simulink model "L400_plant"  (R2022b)
settings: Solver=VariableStepAuto  StartTime=0.0  StopTime=10.0  RelTol=1e-3
InitFcn:
  | L400_init
values from neighbouring files (symbols this model uses):
  db = read_aerody_base('L400气动力数据库.V1.20241219.txt')    [plot_aerody_base.m]
undefined symbols (not defined in the file or in its folder): Earth, Im0, Jm, Kd, Ke, Lm, Rm, WGS84
libraries: aerolibasang x2, aerolib6dof2 x1, matrix_library x1
settings Model: Creator=CETCA  LastModifiedBy=CETCA

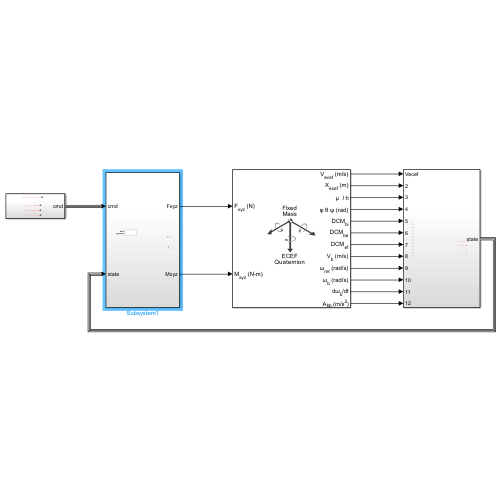
[thumbnail: Simulink's stored preview of the top-level diagram]
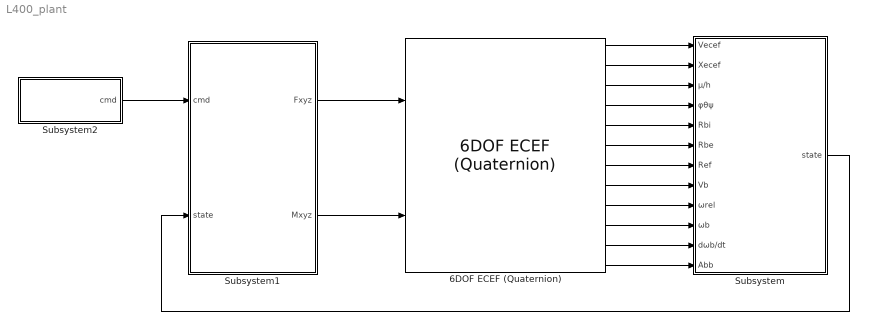
== system L400_plant ==
  6DOF ECEF (Quaternion) : aerolib6dof2/6DOF ECEF (Quaternion)  units=Metric (MKS)  mtype=Fixed  xg_0=[0 0 0]  Vm_0=[0 0 0]  eul_0=[0 0 0]  pm_0=[0 0 0]  mass_0=1.0  mass_e=0.5  mass_f=2.0  inertia=eye(3)  inertia_e=eye(3)  inertia_f=2*eye(3)  vre_flag=on  abi_flag=off  ptype=Earth (WGS84)  R=6378137  F=1/298.257223563  w_E=7292115e-11  angle_in=Internal  LG0=0  quat_statename=''  pm_statename=''  Vm_statename=''  posECEF_statename=''  posECI_statename=''  LG_statename=''  mass_statename=''
  Subsystem : Subsystem
  Subsystem1 : Subsystem
  Subsystem2 : Subsystem
  wires:
  Subsystem/1(state) -> Subsystem1/2(state)
  Subsystem1/1(Fxyz) -> 6DOF ECEF (Quaternion)/1
  Subsystem1/2(Mxyz) -> 6DOF ECEF (Quaternion)/2
  Subsystem2/1(cmd) -> Subsystem1/1(cmd)
  6DOF ECEF (Quaternion)/1 -> Subsystem/1(Vecef)
  6DOF ECEF (Quaternion)/2 -> Subsystem/2(Xecef)
  6DOF ECEF (Quaternion)/3 -> Subsystem/3(μ/h)
  6DOF ECEF (Quaternion)/4 -> Subsystem/4(φθψ)
  6DOF ECEF (Quaternion)/5 -> Subsystem/5(Rbi)
  6DOF ECEF (Quaternion)/6 -> Subsystem/6(Rbe)
  6DOF ECEF (Quaternion)/7 -> Subsystem/7(Ref)
  6DOF ECEF (Quaternion)/8 -> Subsystem/8(Vb)
  6DOF ECEF (Quaternion)/9 -> Subsystem/9(ωrel)
  6DOF ECEF (Quaternion)/10 -> Subsystem/10(ωb)
  6DOF ECEF (Quaternion)/11 -> Subsystem/11(dωb/dt)
  6DOF ECEF (Quaternion)/12 -> Subsystem/12(Abb)

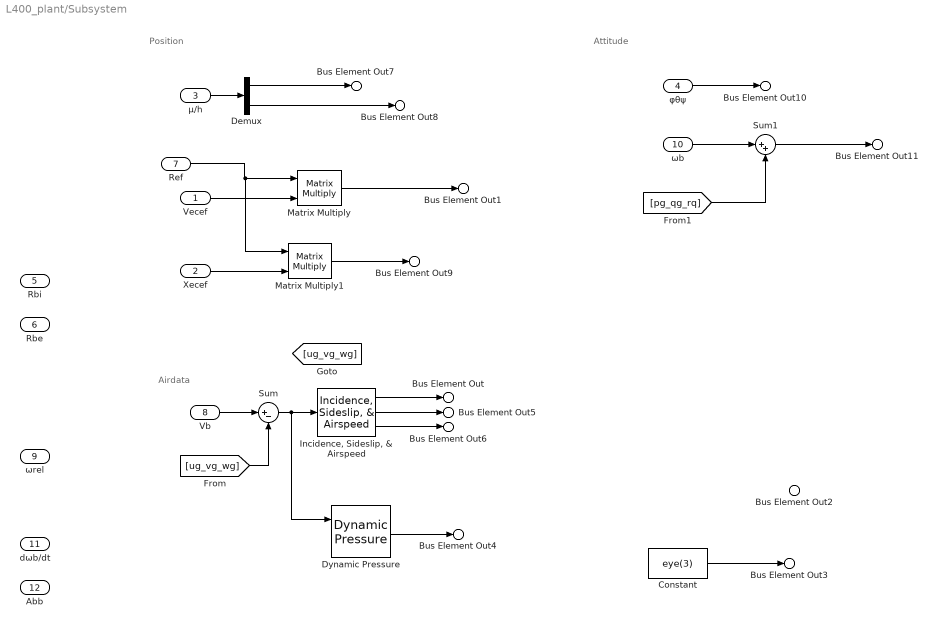
== system L400_plant/Subsystem ==
  note: Attitude
  note: Airdata
  note: Position
  Vecef : Inport
  Xecef : Inport  Port=2
  μ/h : Inport  Port=3
  φθψ : Inport  Port=4
  Rbi : Inport  Port=5
  Rbe : Inport  Port=6
  Ref : Inport  Port=7
  Vb : Inport  Port=8
  ωrel : Inport  Port=9
  ωb : Inport  Port=10
  dωb/dt : Inport  Port=11
  Abb : Inport  Port=12
  Constant : Constant  Value=eye(3)
  Demux : Demux  Outputs=[2 1]
  Dynamic Pressure : aerolibasang/Dynamic Pressure
  "Incidence, Sideslip, & Airspeed" : aerolibasang/Incidence, Sideslip, & Airspeed
  Matrix Multiply : Product  Multiplication=Matrix(*)
  Matrix Multiply1 : Product  Multiplication=Matrix(*)
  Sum : Sum  Inputs=|+-
  Sum1 : Sum  Inputs=|++
  Bus Element Out : Outport  PortName=state  Element=alpha
  Bus Element Out1 : Outport  PortName=state  Element=vn_ve_vd
  Bus Element Out2 : Outport  PortName=state  Element=height
  Bus Element Out3 : Outport  PortName=state  Element=Rbw
  Bus Element Out4 : Outport  PortName=state  Element=qbar
  Bus Element Out5 : Outport  PortName=state  Element=beta
  Bus Element Out6 : Outport  PortName=state  Element=airspeed
  Bus Element Out7 : Outport  PortName=state  Element=lat_lon
  Bus Element Out8 : Outport  PortName=state  Element=alt
  Bus Element Out9 : Outport  PortName=state  Element=pn_pe_pd
  Bus Element Out10 : Outport  PortName=state  Element=phi_theta_psi
  Bus Element Out11 : Outport  PortName=state  Element=p_q_r
  wires:
  Matrix Multiply/1 -> Bus Element Out1/1
  "Incidence, Sideslip, & Airspeed"/1 -> Bus Element Out/1
  Constant/1 -> Bus Element Out3/1
  Vecef/1 -> Matrix Multiply/2
  Ref/1 -> Matrix Multiply1/1, Matrix Multiply/1
  Vb/1 -> Sum/1
  Sum/1 -> Dynamic Pressure/1, "Incidence, Sideslip, & Airspeed"/1
  "Incidence, Sideslip, & Airspeed"/2 -> Bus Element Out5/1
  "Incidence, Sideslip, & Airspeed"/3 -> Bus Element Out6/1
  [ug_vg_wg] -> Sum/2
  Dynamic Pressure/1 -> Bus Element Out4/1
  μ/h/1 -> Demux/1
  Demux/1 -> Bus Element Out7/1
  Demux/2 -> Bus Element Out8/1
  Xecef/1 -> Matrix Multiply1/2
  Matrix Multiply1/1 -> Bus Element Out9/1
  φθψ/1 -> Bus Element Out10/1
  ωb/1 -> Sum1/1
  Sum1/1 -> Bus Element Out11/1
  [pg_qg_rq] -> Sum1/2

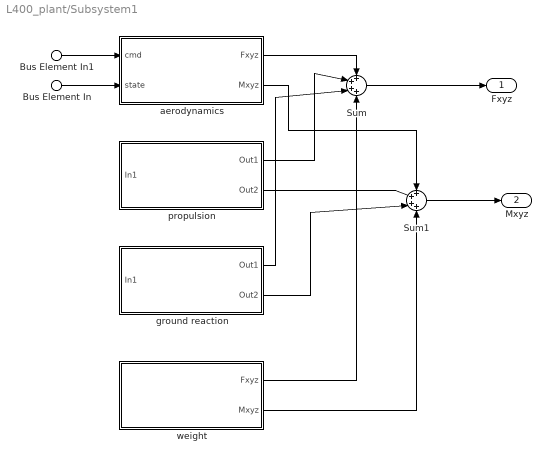
== system L400_plant/Subsystem1 ==
  Bus Element In1 : Inport  PortName=cmd
  Bus Element In : Inport  Port=2  PortName=state
  Sum : Sum  Inputs=4
  Sum1 : Sum  Inputs=4
  aerodynamics : Subsystem
  ground reaction : Subsystem
  propulsion : Subsystem
  weight : Subsystem
  Fxyz : Outport
  Mxyz : Outport  Port=2
  wires:
  Bus Element In/1 -> aerodynamics/2(state)
  Bus Element In1/1 -> aerodynamics/1(cmd)
  propulsion/2(Out2) -> Sum1/2
  aerodynamics/1(Fxyz) -> Sum/1
  propulsion/1(Out1) -> Sum/2
  aerodynamics/2(Mxyz) -> Sum1/1
  Sum1/1 -> Mxyz/1
  Sum/1 -> Fxyz/1
  ground reaction/1(Out1) -> Sum/3
  ground reaction/2(Out2) -> Sum1/3
  weight/1(Fxyz) -> Sum/4
  weight/2(Mxyz) -> Sum1/4

== system L400_plant/Subsystem2 ==
  Bus Element Out : Outport  PortName=cmd  Element=df
  Bus Element Out1 : Outport  PortName=cmd  Element=da
  Bus Element Out2 : Outport  PortName=cmd  Element=dr
  Bus Element Out3 : Outport  PortName=cmd  Element=de
  wires:
  ? -> Bus Element Out/1
  ? -> Bus Element Out1/1
  ? -> Bus Element Out3/1
  ? -> Bus Element Out2/1

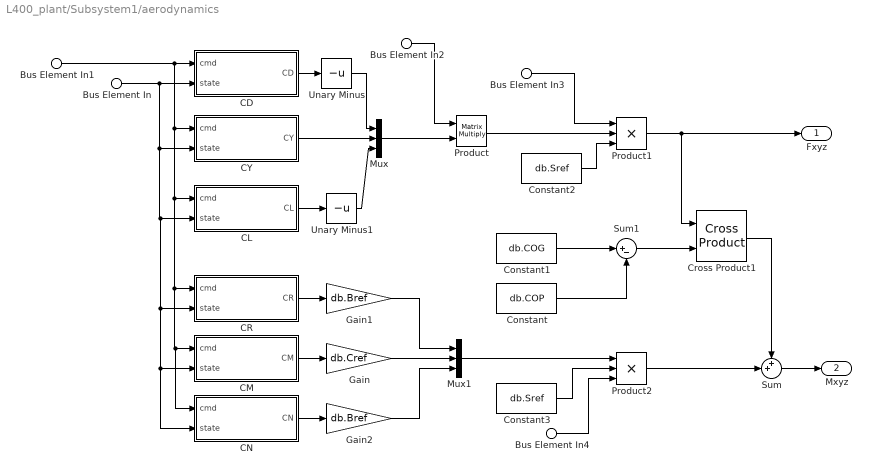
== system L400_plant/Subsystem1/aerodynamics ==
  Bus Element In1 : Inport  PortName=cmd
  Bus Element In : Inport  Port=2  PortName=state
  Bus Element In2 : Inport  Port=2  PortName=state  Element=Rbw
  Bus Element In3 : Inport  Port=2  PortName=state  Element=qbar
  Bus Element In4 : Inport  Port=2  PortName=state  Element=qbar
  CD : Subsystem
  CL : Subsystem
  CM : Subsystem
  CN : Subsystem
  CR : Subsystem
  CY : Subsystem
  Constant : Constant  Value=db.COP
  Constant1 : Constant  Value=db.COG
  Constant2 : Constant  Value=db.Sref
  Constant3 : Constant  Value=db.Sref
  Cross Product1 : matrix_library/Cross Product
  Gain : Gain  Gain=db.Cref
  Gain1 : Gain  Gain=db.Bref
  Gain2 : Gain  Gain=db.Bref
  Mux : Mux  Inputs=3
  Mux1 : Mux  Inputs=3
  Product : Product  Multiplication=Matrix(*)
  Product1 : Product  Inputs=3
  Product2 : Product  Inputs=3
  Sum : Sum  Inputs=++|
  Sum1 : Sum  Inputs=|+-
  Unary Minus : UnaryMinus
  Unary Minus1 : UnaryMinus
  Fxyz : Outport
  Mxyz : Outport  Port=2
  wires:
  Bus Element In1/1 -> CN/1(cmd), CM/1(cmd), CR/1(cmd), CL/1(cmd), CY/1(cmd), CD/1(cmd)
  Bus Element In/1 -> CN/2(state), CM/2(state), CR/2(state), CL/2(state), CY/2(state), CD/2(state)
  Mux/1 -> Product/2
  CD/1(CD) -> Unary Minus/1
  CY/1(CY) -> Mux/2
  CL/1(CL) -> Unary Minus1/1
  Unary Minus/1 -> Mux/1
  Unary Minus1/1 -> Mux/3
  Product/1 -> Product1/2
  Bus Element In2/1 -> Product/1
  CM/1(CM) -> Gain/1
  CR/1(CR) -> Gain1/1
  CN/1(CN) -> Gain2/1
  Mux1/1 -> Product2/1
  Sum/1 -> Mxyz/1
  Cross Product1/1 -> Sum/1
  Constant1/1 -> Sum1/1
  Constant/1 -> Sum1/2
  Product1/1 -> Cross Product1/1, Fxyz/1
  Bus Element In3/1 -> Product1/1
  Constant2/1 -> Product1/3
  Product2/1 -> Sum/2
  Bus Element In4/1 -> Product2/3
  Constant3/1 -> Product2/2
  Gain/1 -> Mux1/2
  Gain1/1 -> Mux1/1
  Gain2/1 -> Mux1/3
  Sum1/1 -> Cross Product1/2

== system L400_plant/Subsystem1/ground reaction ==
  In1 : Inport
  Out1 : Outport
  Out2 : Outport  Port=2

== system L400_plant/Subsystem1/propulsion ==
  In1 : Inport
  Subsystem : Subsystem
  Out1 : Outport
  Out2 : Outport  Port=2

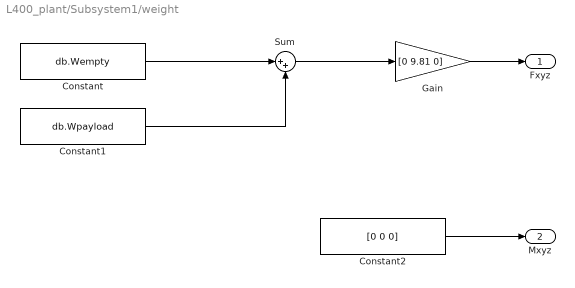
== system L400_plant/Subsystem1/weight ==
  Constant : Constant  Value=db.Wempty
  Constant1 : Constant  Value=db.Wpayload
  Constant2 : Constant  Value=[0 0 0]
  Gain : Gain  Gain=[0 9.81 0]
  Sum : Sum  Inputs=|++
  Fxyz : Outport
  Mxyz : Outport  Port=2
  wires:
  Constant/1 -> Sum/1
  Constant1/1 -> Sum/2
  Sum/1 -> Gain/1
  Gain/1 -> Fxyz/1
  Constant2/1 -> Mxyz/1

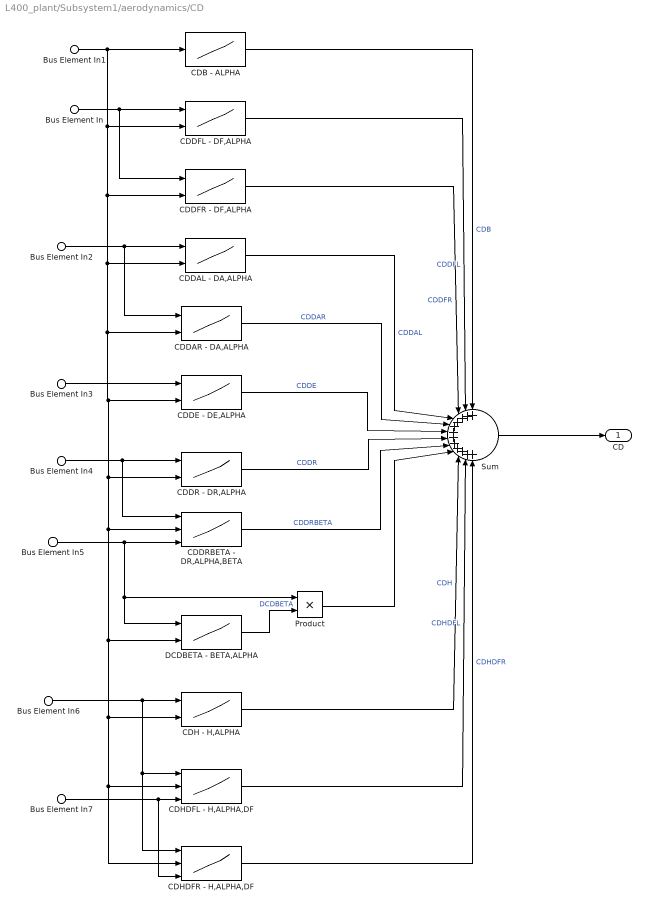
== system L400_plant/Subsystem1/aerodynamics/CD ==
  Bus Element In : Inport  PortName=cmd  Element=df
  Bus Element In7 : Inport  PortName=cmd  Element=df
  Bus Element In2 : Inport  PortName=cmd  Element=da
  Bus Element In3 : Inport  PortName=cmd  Element=de
  Bus Element In4 : Inport  PortName=cmd  Element=dr
  Bus Element In1 : Inport  Port=2  PortName=state  Element=alpha
  Bus Element In5 : Inport  Port=2  PortName=state  Element=vn_ve_vd
  Bus Element In6 : Inport  Port=2  PortName=state  Element=height
  CDB - ALPHA : Lookup_n-D  NumberOfTableDimensions=1  BreakpointsForDimension1=db.VALPHA  Table=db.CDB  InternalRulePriority=Speed  RndMeth=Simplest
  CDDAL - DA,ALPHA : Lookup_n-D  BreakpointsForDimension1=db.VDA  BreakpointsForDimension2=db.VALPHA  Table=db.CDDAL  InternalRulePriority=Speed  RndMeth=Simplest
      settings: InputPortMap=u0,u1
  CDDAR - DA,ALPHA : Lookup_n-D  BreakpointsForDimension1=db.VDA  BreakpointsForDimension2=db.VALPHA  Table=db.CDDAR  InternalRulePriority=Speed  RndMeth=Simplest
      settings: InputPortMap=u0,u1
  CDDE - DE,ALPHA : Lookup_n-D  BreakpointsForDimension1=db.VDE  BreakpointsForDimension2=db.VALPHA  Table=db.CDDE  InternalRulePriority=Speed  RndMeth=Simplest
      settings: InputPortMap=u0,u1
  CDDFL - DF,ALPHA : Lookup_n-D  BreakpointsForDimension1=db.VDF  BreakpointsForDimension2=db.VALPHA  Table=db.CDDFL  InternalRulePriority=Speed  RndMeth=Simplest
      settings: InputPortMap=u0,u1
  CDDFR - DF,ALPHA : Lookup_n-D  BreakpointsForDimension1=db.VDF  BreakpointsForDimension2=db.VALPHA  Table=db.CDDFR  InternalRulePriority=Speed  RndMeth=Simplest
      settings: InputPortMap=u0,u1
  CDDR - DR,ALPHA : Lookup_n-D  BreakpointsForDimension1=db.VDR  BreakpointsForDimension2=db.VALPHA  Table=db.CDDR  InternalRulePriority=Speed  RndMeth=Simplest
      settings: InputPortMap=u0,u1
  CDDRBETA - DR,ALPHA,BETA : Lookup_n-D  NumberOfTableDimensions=3  BreakpointsForDimension1=db.VDR  BreakpointsForDimension2=db.VALPHA  BreakpointsForDimension3=db.VBETA  Table=db.CDDRBETA  InternalRulePriority=Speed  RndMeth=Simplest
      settings: InputPortMap=u0,u1,u2
  CDH - H,ALPHA : Lookup_n-D  BreakpointsForDimension1=db.VH  BreakpointsForDimension2=db.VALPHA  Table=db.CDH  InternalRulePriority=Speed  RndMeth=Simplest
      settings: InputPortMap=u0,u1
  CDHDFL - H,ALPHA,DF : Lookup_n-D  NumberOfTableDimensions=3  BreakpointsForDimension1=db.VH  BreakpointsForDimension2=db.VALPHA  BreakpointsForDimension3=db.VDF  Table=db.CDHDFL  InternalRulePriority=Speed  RndMeth=Simplest
      settings: InputPortMap=u0,u1,u2
  CDHDFR - H,ALPHA,DF : Lookup_n-D  NumberOfTableDimensions=3  BreakpointsForDimension1=db.VH  BreakpointsForDimension2=db.VALPHA  BreakpointsForDimension3=db.VDF  Table=db.CDHDFR  InternalRulePriority=Speed  RndMeth=Simplest
      settings: InputPortMap=u0,u1,u2
  DCDBETA - BETA,ALPHA : Lookup_n-D  BreakpointsForDimension1=db.VBETA  BreakpointsForDimension2=db.VALPHA  Table=db.DCDBETA  InternalRulePriority=Speed  RndMeth=Simplest
      settings: InputPortMap=u0,u1
  Product : Product
  Sum : Sum  Inputs=12
  CD : Outport
  wires:
  CDB - ALPHA/1 -> Sum/1  "CDB"
  Bus Element In1/1 -> CDDAR - DA,ALPHA/2, CDDR - DR,ALPHA/2, CDDRBETA - DR,ALPHA,BETA/2, DCDBETA - BETA,ALPHA/2, CDHDFL - H,ALPHA,DF/2, CDHDFR - H,ALPHA,DF/2, CDH - H,ALPHA/2, CDDE - DE,ALPHA/2, CDDAL - DA,ALPHA/2, CDDFR - DF,ALPHA/2, CDDFL - DF,ALPHA/2, CDB - ALPHA/1
  CDDFL - DF,ALPHA/1 -> Sum/2  "CDDFL"
  Bus Element In/1 -> CDDFR - DF,ALPHA/1, CDDFL - DF,ALPHA/1
  CDDFR - DF,ALPHA/1 -> Sum/3  "CDDFR"
  CDDAL - DA,ALPHA/1 -> Sum/4  "CDDAL"
  Bus Element In2/1 -> CDDAR - DA,ALPHA/1, CDDAL - DA,ALPHA/1
  CDDAR - DA,ALPHA/1 -> Sum/5  "CDDAR"
  CDDE - DE,ALPHA/1 -> Sum/6  "CDDE"
  Bus Element In3/1 -> CDDE - DE,ALPHA/1
  CDDR - DR,ALPHA/1 -> Sum/7  "CDDR"
  Bus Element In4/1 -> CDDRBETA - DR,ALPHA,BETA/1, CDDR - DR,ALPHA/1
  CDDRBETA - DR,ALPHA,BETA/1 -> Sum/8  "CDDRBETA"
  Bus Element In5/1 -> Product/1, DCDBETA - BETA,ALPHA/1, CDDRBETA - DR,ALPHA,BETA/3
  DCDBETA - BETA,ALPHA/1 -> Product/2  "DCDBETA"
  Product/1 -> Sum/9
  CDH - H,ALPHA/1 -> Sum/10  "CDH"
  Bus Element In6/1 -> CDHDFR - H,ALPHA,DF/1, CDHDFL - H,ALPHA,DF/1, CDH - H,ALPHA/1
  CDHDFL - H,ALPHA,DF/1 -> Sum/11  "CDHDFL"
  Bus Element In7/1 -> CDHDFR - H,ALPHA,DF/3, CDHDFL - H,ALPHA,DF/3
  CDHDFR - H,ALPHA,DF/1 -> Sum/12  "CDHDFR"
  Sum/1 -> CD/1

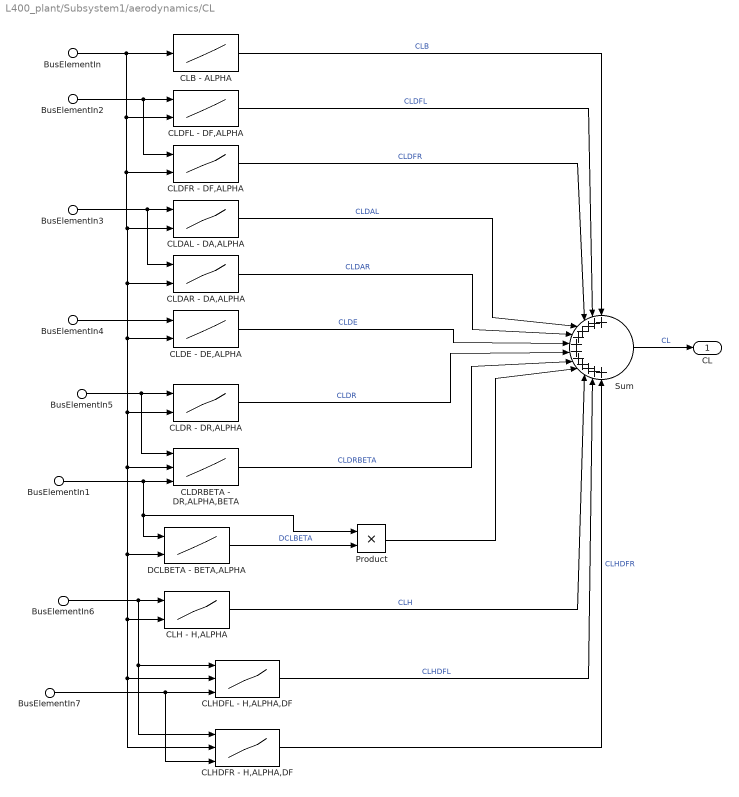
== system L400_plant/Subsystem1/aerodynamics/CL ==
  BusElementIn2 : Inport  PortName=cmd  Element=df
  BusElementIn7 : Inport  PortName=cmd  Element=df
  BusElementIn3 : Inport  PortName=cmd  Element=da
  BusElementIn4 : Inport  PortName=cmd  Element=de
  BusElementIn5 : Inport  PortName=cmd  Element=dr
  BusElementIn : Inport  Port=2  PortName=state  Element=alpha
  BusElementIn1 : Inport  Port=2  PortName=state  Element=vn_ve_vd
  BusElementIn6 : Inport  Port=2  PortName=state  Element=height
  CLB - ALPHA : Lookup_n-D  NumberOfTableDimensions=1  BreakpointsForDimension1=db.VALPHA  Table=db.CLB  InternalRulePriority=Speed  RndMeth=Simplest
  CLDAL - DA,ALPHA : Lookup_n-D  BreakpointsForDimension1=db.VDA  BreakpointsForDimension2=db.VALPHA  Table=db.CLDAL  InternalRulePriority=Speed  RndMeth=Simplest
      settings: InputPortMap=u0,u1
  CLDAR - DA,ALPHA : Lookup_n-D  BreakpointsForDimension1=db.VDA  BreakpointsForDimension2=db.VALPHA  Table=db.CLDAR  InternalRulePriority=Speed  RndMeth=Simplest
      settings: InputPortMap=u0,u1
  CLDE - DE,ALPHA : Lookup_n-D  BreakpointsForDimension1=db.VDE  BreakpointsForDimension2=db.VALPHA  Table=db.CLDE  InternalRulePriority=Speed  RndMeth=Simplest
      settings: InputPortMap=u0,u1
  CLDFL - DF,ALPHA : Lookup_n-D  BreakpointsForDimension1=db.VDF  BreakpointsForDimension2=db.VALPHA  Table=db.CLDFL  InternalRulePriority=Speed  RndMeth=Simplest
      settings: InputPortMap=u0,u1
  CLDFR - DF,ALPHA : Lookup_n-D  BreakpointsForDimension1=db.VDF  BreakpointsForDimension2=db.VALPHA  Table=db.CLDFR  InternalRulePriority=Speed  RndMeth=Simplest
      settings: InputPortMap=u0,u1
  CLDR - DR,ALPHA : Lookup_n-D  BreakpointsForDimension1=db.VDR  BreakpointsForDimension2=db.VALPHA  Table=db.CLDR  InternalRulePriority=Speed  RndMeth=Simplest
      settings: InputPortMap=u0,u1
  CLDRBETA - DR,ALPHA,BETA : Lookup_n-D  NumberOfTableDimensions=3  BreakpointsForDimension1=db.VDR  BreakpointsForDimension2=db.VALPHA  BreakpointsForDimension3=db.VBETA  Table=db.CLDRBETA  InternalRulePriority=Speed  RndMeth=Simplest
      settings: InputPortMap=u0,u1,u2
  CLH - H,ALPHA : Lookup_n-D  BreakpointsForDimension1=db.VH  BreakpointsForDimension2=db.VALPHA  BreakpointsForDimension3=db.VBETA  Table=db.CLH  InternalRulePriority=Speed  RndMeth=Simplest
      settings: InputPortMap=u0,u1
  CLHDFL - H,ALPHA,DF : Lookup_n-D  NumberOfTableDimensions=3  BreakpointsForDimension1=db.VH  BreakpointsForDimension2=db.VALPHA  BreakpointsForDimension3=db.VDF  Table=db.CLHDFL  InternalRulePriority=Speed  RndMeth=Simplest
      settings: InputPortMap=u0,u1,u2
  CLHDFR - H,ALPHA,DF : Lookup_n-D  NumberOfTableDimensions=3  BreakpointsForDimension1=db.VH  BreakpointsForDimension2=db.VALPHA  BreakpointsForDimension3=db.VDF  Table=db.CLHDFL  InternalRulePriority=Speed  RndMeth=Simplest
      settings: InputPortMap=u0,u1,u2
  DCLBETA - BETA,ALPHA : Lookup_n-D  BreakpointsForDimension1=db.VBETA  BreakpointsForDimension2=db.VALPHA  BreakpointsForDimension3=db.VBETA  Table=db.DCLBETA  InternalRulePriority=Speed  RndMeth=Simplest
      settings: InputPortMap=u0,u1
  Product : Product
  Sum : Sum  Inputs=12
  CL : Outport
  wires:
  BusElementIn/1 -> DCLBETA - BETA,ALPHA/2, CLHDFR - H,ALPHA,DF/2, CLHDFL - H,ALPHA,DF/2, CLH - H,ALPHA/2, CLDRBETA - DR,ALPHA,BETA/2, CLDR - DR,ALPHA/2, CLDE - DE,ALPHA/2, CLDAR - DA,ALPHA/2, CLDAL - DA,ALPHA/2, CLDFR - DF,ALPHA/2, CLDFL - DF,ALPHA/2, CLB - ALPHA/1
  CLB - ALPHA/1 -> Sum/1  "CLB"
  BusElementIn2/1 -> CLDFR - DF,ALPHA/1, CLDFL - DF,ALPHA/1
  CLDFL - DF,ALPHA/1 -> Sum/2  "CLDFL"
  CLDFR - DF,ALPHA/1 -> Sum/3  "CLDFR"
  CLDAL - DA,ALPHA/1 -> Sum/4  "CLDAL"
  BusElementIn3/1 -> CLDAR - DA,ALPHA/1, CLDAL - DA,ALPHA/1
  CLDAR - DA,ALPHA/1 -> Sum/5  "CLDAR"
  BusElementIn4/1 -> CLDE - DE,ALPHA/1
  CLDE - DE,ALPHA/1 -> Sum/6  "CLDE"
  CLDR - DR,ALPHA/1 -> Sum/7  "CLDR"
  BusElementIn5/1 -> CLDRBETA - DR,ALPHA,BETA/1, CLDR - DR,ALPHA/1
  Sum/1 -> CL/1  "CL"
  CLDRBETA - DR,ALPHA,BETA/1 -> Sum/8  "CLDRBETA"
  BusElementIn1/1 -> Product/1, DCLBETA - BETA,ALPHA/1, CLDRBETA - DR,ALPHA,BETA/3
  DCLBETA - BETA,ALPHA/1 -> Product/2  "DCLBETA"
  Product/1 -> Sum/9
  CLH - H,ALPHA/1 -> Sum/10  "CLH"
  BusElementIn6/1 -> CLHDFR - H,ALPHA,DF/1, CLHDFL - H,ALPHA,DF/1, CLH - H,ALPHA/1
  CLHDFL - H,ALPHA,DF/1 -> Sum/11  "CLHDFL"
  BusElementIn7/1 -> CLHDFR - H,ALPHA,DF/3, CLHDFL - H,ALPHA,DF/3
  CLHDFR - H,ALPHA,DF/1 -> Sum/12  "CLHDFR"

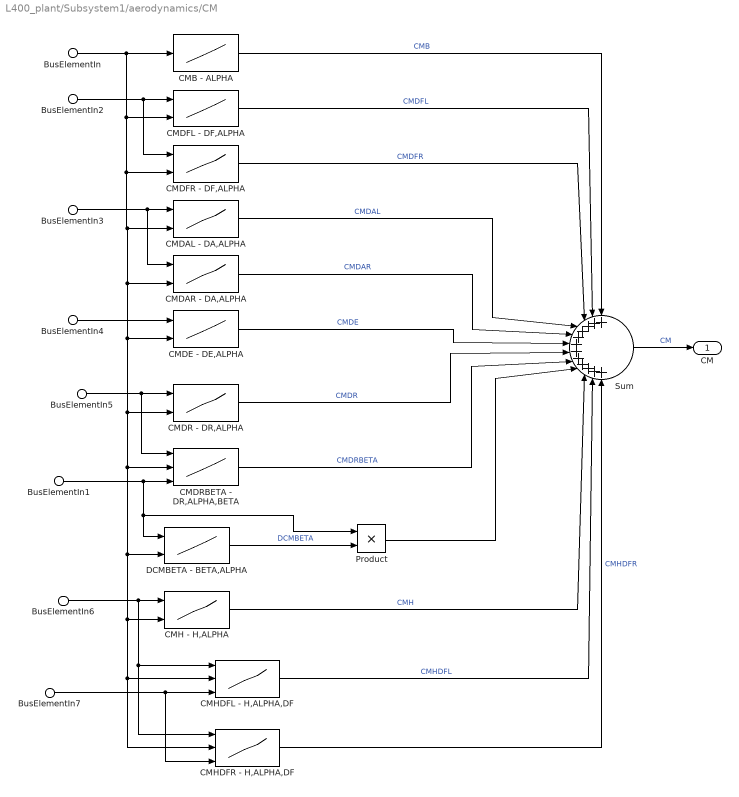
== system L400_plant/Subsystem1/aerodynamics/CM ==
  BusElementIn2 : Inport  PortName=cmd  Element=df
  BusElementIn7 : Inport  PortName=cmd  Element=df
  BusElementIn3 : Inport  PortName=cmd  Element=da
  BusElementIn4 : Inport  PortName=cmd  Element=de
  BusElementIn5 : Inport  PortName=cmd  Element=dr
  BusElementIn : Inport  Port=2  PortName=state  Element=alpha
  BusElementIn1 : Inport  Port=2  PortName=state  Element=vn_ve_vd
  BusElementIn6 : Inport  Port=2  PortName=state  Element=height
  CMB - ALPHA : Lookup_n-D  NumberOfTableDimensions=1  BreakpointsForDimension1=db.VALPHA  Table=db.CMB  InternalRulePriority=Speed  RndMeth=Simplest
  CMDAL - DA,ALPHA : Lookup_n-D  BreakpointsForDimension1=db.VDA  BreakpointsForDimension2=db.VALPHA  Table=db.CMDAL  InternalRulePriority=Speed  RndMeth=Simplest
      settings: InputPortMap=u0,u1
  CMDAR - DA,ALPHA : Lookup_n-D  BreakpointsForDimension1=db.VDA  BreakpointsForDimension2=db.VALPHA  Table=db.CMDAR  InternalRulePriority=Speed  RndMeth=Simplest
      settings: InputPortMap=u0,u1
  CMDE - DE,ALPHA : Lookup_n-D  BreakpointsForDimension1=db.VDE  BreakpointsForDimension2=db.VALPHA  Table=db.CMDE  InternalRulePriority=Speed  RndMeth=Simplest
      settings: InputPortMap=u0,u1
  CMDFL - DF,ALPHA : Lookup_n-D  BreakpointsForDimension1=db.VDF  BreakpointsForDimension2=db.VALPHA  Table=db.CMDFL  InternalRulePriority=Speed  RndMeth=Simplest
      settings: InputPortMap=u0,u1
  CMDFR - DF,ALPHA : Lookup_n-D  BreakpointsForDimension1=db.VDF  BreakpointsForDimension2=db.VALPHA  Table=db.CMDFR  InternalRulePriority=Speed  RndMeth=Simplest
      settings: InputPortMap=u0,u1
  CMDR - DR,ALPHA : Lookup_n-D  BreakpointsForDimension1=db.VDR  BreakpointsForDimension2=db.VALPHA  Table=db.CMDR  InternalRulePriority=Speed  RndMeth=Simplest
      settings: InputPortMap=u0,u1
  CMDRBETA - DR,ALPHA,BETA : Lookup_n-D  NumberOfTableDimensions=3  BreakpointsForDimension1=db.VDR  BreakpointsForDimension2=db.VALPHA  BreakpointsForDimension3=db.VBETA  Table=db.CMDRBETA  InternalRulePriority=Speed  RndMeth=Simplest
      settings: InputPortMap=u0,u1,u2
  CMH - H,ALPHA : Lookup_n-D  BreakpointsForDimension1=db.VH  BreakpointsForDimension2=db.VALPHA  BreakpointsForDimension3=db.VBETA  Table=db.CMH  InternalRulePriority=Speed  RndMeth=Simplest
      settings: InputPortMap=u0,u1
  CMHDFL - H,ALPHA,DF : Lookup_n-D  NumberOfTableDimensions=3  BreakpointsForDimension1=db.VH  BreakpointsForDimension2=db.VALPHA  BreakpointsForDimension3=db.VDF  Table=db.CMHDFL  InternalRulePriority=Speed  RndMeth=Simplest
      settings: InputPortMap=u0,u1,u2
  CMHDFR - H,ALPHA,DF : Lookup_n-D  NumberOfTableDimensions=3  BreakpointsForDimension1=db.VH  BreakpointsForDimension2=db.VALPHA  BreakpointsForDimension3=db.VDF  Table=db.CMHDFR  InternalRulePriority=Speed  RndMeth=Simplest
      settings: InputPortMap=u0,u1,u2
  DCMBETA - BETA,ALPHA : Lookup_n-D  BreakpointsForDimension1=db.VBETA  BreakpointsForDimension2=db.VALPHA  BreakpointsForDimension3=db.VBETA  Table=db.DCMBETA  InternalRulePriority=Speed  RndMeth=Simplest
      settings: InputPortMap=u0,u1
  Product : Product
  Sum : Sum  Inputs=12
  CM : Outport
  wires:
  CMHDFR - H,ALPHA,DF/1 -> Sum/12  "CMHDFR"
  BusElementIn7/1 -> CMHDFL - H,ALPHA,DF/3, CMHDFR - H,ALPHA,DF/3
  CMHDFL - H,ALPHA,DF/1 -> Sum/11  "CMHDFL"
  BusElementIn6/1 -> CMH - H,ALPHA/1, CMHDFL - H,ALPHA,DF/1, CMHDFR - H,ALPHA,DF/1
  CMH - H,ALPHA/1 -> Sum/10  "CMH"
  Product/1 -> Sum/9
  DCMBETA - BETA,ALPHA/1 -> Product/2  "DCMBETA"
  BusElementIn1/1 -> CMDRBETA - DR,ALPHA,BETA/3, DCMBETA - BETA,ALPHA/1, Product/1
  CMDRBETA - DR,ALPHA,BETA/1 -> Sum/8  "CMDRBETA"
  Sum/1 -> CM/1  "CM"
  BusElementIn5/1 -> CMDR - DR,ALPHA/1, CMDRBETA - DR,ALPHA,BETA/1
  CMDR - DR,ALPHA/1 -> Sum/7  "CMDR"
  CMDE - DE,ALPHA/1 -> Sum/6  "CMDE"
  BusElementIn4/1 -> CMDE - DE,ALPHA/1
  CMDAR - DA,ALPHA/1 -> Sum/5  "CMDAR"
  BusElementIn3/1 -> CMDAL - DA,ALPHA/1, CMDAR - DA,ALPHA/1
  CMDAL - DA,ALPHA/1 -> Sum/4  "CMDAL"
  CMDFR - DF,ALPHA/1 -> Sum/3  "CMDFR"
  CMDFL - DF,ALPHA/1 -> Sum/2  "CMDFL"
  BusElementIn2/1 -> CMDFL - DF,ALPHA/1, CMDFR - DF,ALPHA/1
  CMB - ALPHA/1 -> Sum/1  "CMB"
  BusElementIn/1 -> CMB - ALPHA/1, CMDFL - DF,ALPHA/2, CMDFR - DF,ALPHA/2, CMDAL - DA,ALPHA/2, CMDAR - DA,ALPHA/2, CMDE - DE,ALPHA/2, CMDR - DR,ALPHA/2, CMDRBETA - DR,ALPHA,BETA/2, CMH - H,ALPHA/2, CMHDFL - H,ALPHA,DF/2, CMHDFR - H,ALPHA,DF/2, DCMBETA - BETA,ALPHA/2

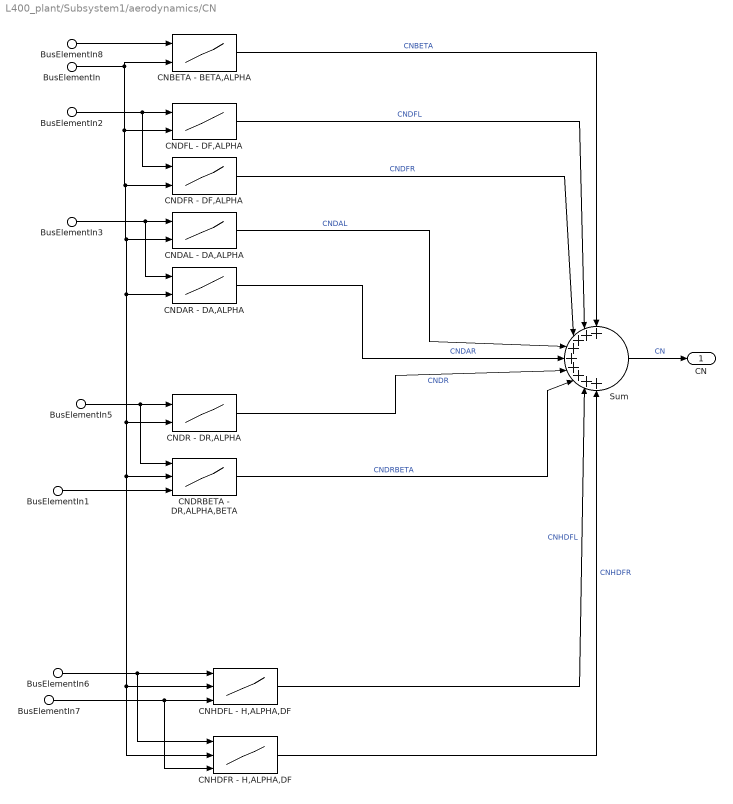
== system L400_plant/Subsystem1/aerodynamics/CN ==
  BusElementIn2 : Inport  PortName=cmd  Element=df
  BusElementIn7 : Inport  PortName=cmd  Element=df
  BusElementIn3 : Inport  PortName=cmd  Element=da
  BusElementIn5 : Inport  PortName=cmd  Element=dr
  BusElementIn : Inport  Port=2  PortName=state  Element=alpha
  BusElementIn6 : Inport  Port=2  PortName=state  Element=height
  BusElementIn1 : Inport  Port=2  PortName=state  Element=vn_ve_vd
  BusElementIn8 : Inport  Port=2  PortName=state  Element=vn_ve_vd
  CNBETA - BETA,ALPHA : Lookup_n-D  BreakpointsForDimension1=db.VBETA  BreakpointsForDimension2=db.VALPHA  Table=db.CNBETA  InternalRulePriority=Speed  RndMeth=Simplest
      settings: InputPortMap=u0,u1
  CNDAL - DA,ALPHA : Lookup_n-D  BreakpointsForDimension1=db.VDA  BreakpointsForDimension2=db.VALPHA  Table=db.CNDAL  InternalRulePriority=Speed  RndMeth=Simplest
      settings: InputPortMap=u0,u1
  CNDAR - DA,ALPHA : Lookup_n-D  BreakpointsForDimension1=db.VDA  BreakpointsForDimension2=db.VALPHA  Table=db.CNDAR  InternalRulePriority=Speed  RndMeth=Simplest
      settings: InputPortMap=u0,u1
  CNDFL - DF,ALPHA : Lookup_n-D  BreakpointsForDimension1=db.VDF  BreakpointsForDimension2=db.VALPHA  Table=db.CNDFL  InternalRulePriority=Speed  RndMeth=Simplest
      settings: InputPortMap=u0,u1
  CNDFR - DF,ALPHA : Lookup_n-D  BreakpointsForDimension1=db.VDF  BreakpointsForDimension2=db.VALPHA  Table=db.CNDFR  InternalRulePriority=Speed  RndMeth=Simplest
      settings: InputPortMap=u0,u1
  CNDR - DR,ALPHA : Lookup_n-D  BreakpointsForDimension1=db.VDR  BreakpointsForDimension2=db.VALPHA  Table=db.CNDR  InternalRulePriority=Speed  RndMeth=Simplest
      settings: InputPortMap=u0,u1
  CNDRBETA - DR,ALPHA,BETA : Lookup_n-D  NumberOfTableDimensions=3  BreakpointsForDimension1=db.VDR  BreakpointsForDimension2=db.VALPHA  BreakpointsForDimension3=db.VBETA  Table=db.CNDRBETA  InternalRulePriority=Speed  RndMeth=Simplest
      settings: InputPortMap=u0,u1,u2
  CNHDFL - H,ALPHA,DF : Lookup_n-D  NumberOfTableDimensions=3  BreakpointsForDimension1=db.VH  BreakpointsForDimension2=db.VALPHA  BreakpointsForDimension3=db.VDF  Table=db.CNHDFL  InternalRulePriority=Speed  RndMeth=Simplest
      settings: InputPortMap=u0,u1,u2
  CNHDFR - H,ALPHA,DF : Lookup_n-D  NumberOfTableDimensions=3  BreakpointsForDimension1=db.VH  BreakpointsForDimension2=db.VALPHA  BreakpointsForDimension3=db.VDF  Table=db.CNHDFR  InternalRulePriority=Speed  RndMeth=Simplest
      settings: InputPortMap=u0,u1,u2
  Sum : Sum  Inputs=9
  CN : Outport
  wires:
  BusElementIn/1 -> CNHDFR - H,ALPHA,DF/2, CNHDFL - H,ALPHA,DF/2, CNDRBETA - DR,ALPHA,BETA/2, CNDR - DR,ALPHA/2, CNDAR - DA,ALPHA/2, CNDAL - DA,ALPHA/2, CNDFR - DF,ALPHA/2, CNDFL - DF,ALPHA/2, CNBETA - BETA,ALPHA/2
  CNBETA - BETA,ALPHA/1 -> Sum/1  "CNBETA"
  BusElementIn2/1 -> CNDFR - DF,ALPHA/1, CNDFL - DF,ALPHA/1
  CNDFL - DF,ALPHA/1 -> Sum/2  "CNDFL"
  CNDFR - DF,ALPHA/1 -> Sum/3  "CNDFR"
  CNDAL - DA,ALPHA/1 -> Sum/4  "CNDAL"
  BusElementIn3/1 -> CNDAR - DA,ALPHA/1, CNDAL - DA,ALPHA/1
  CNDAR - DA,ALPHA/1 -> Sum/5  "CNDAR"
  CNDR - DR,ALPHA/1 -> Sum/6  "CNDR"
  BusElementIn5/1 -> CNDRBETA - DR,ALPHA,BETA/1, CNDR - DR,ALPHA/1
  Sum/1 -> CN/1  "CN"
  CNDRBETA - DR,ALPHA,BETA/1 -> Sum/7  "CNDRBETA"
  BusElementIn1/1 -> CNDRBETA - DR,ALPHA,BETA/3
  BusElementIn6/1 -> CNHDFR - H,ALPHA,DF/1, CNHDFL - H,ALPHA,DF/1
  CNHDFL - H,ALPHA,DF/1 -> Sum/8  "CNHDFL"
  BusElementIn7/1 -> CNHDFR - H,ALPHA,DF/3, CNHDFL - H,ALPHA,DF/3
  CNHDFR - H,ALPHA,DF/1 -> Sum/9  "CNHDFR"
  BusElementIn8/1 -> CNBETA - BETA,ALPHA/1

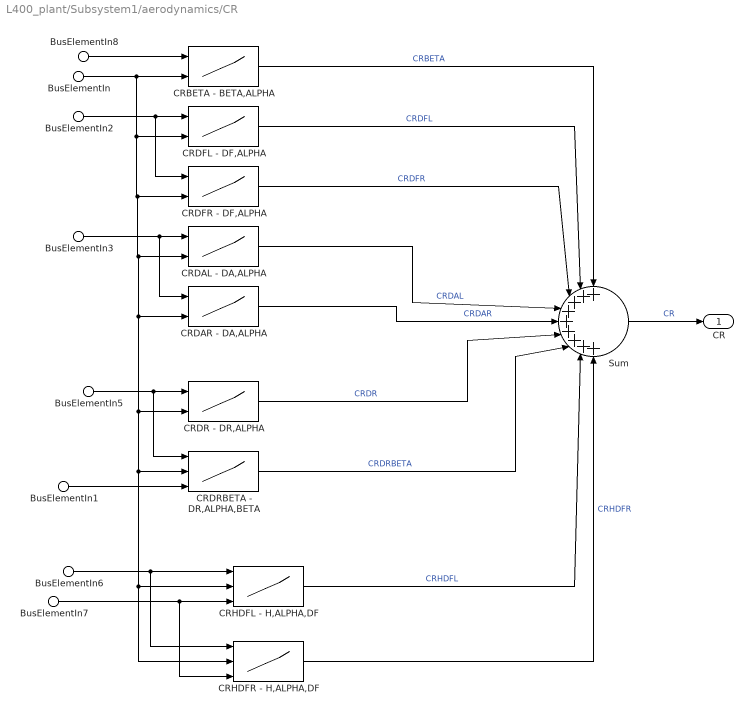
== system L400_plant/Subsystem1/aerodynamics/CR ==
  BusElementIn2 : Inport  PortName=cmd  Element=df
  BusElementIn7 : Inport  PortName=cmd  Element=df
  BusElementIn3 : Inport  PortName=cmd  Element=da
  BusElementIn5 : Inport  PortName=cmd  Element=dr
  BusElementIn : Inport  Port=2  PortName=state  Element=alpha
  BusElementIn6 : Inport  Port=2  PortName=state  Element=height
  BusElementIn1 : Inport  Port=2  PortName=state  Element=vn_ve_vd
  BusElementIn8 : Inport  Port=2  PortName=state  Element=vn_ve_vd
  CRBETA - BETA,ALPHA : Lookup_n-D  BreakpointsForDimension1=db.VBETA  BreakpointsForDimension2=db.VALPHA  Table=db.CRBETA  InternalRulePriority=Speed  RndMeth=Simplest
      settings: InputPortMap=u0,u1
  CRDAL - DA,ALPHA : Lookup_n-D  BreakpointsForDimension1=db.VDA  BreakpointsForDimension2=db.VALPHA  Table=db.CRDAL  InternalRulePriority=Speed  RndMeth=Simplest
      settings: InputPortMap=u0,u1
  CRDAR - DA,ALPHA : Lookup_n-D  BreakpointsForDimension1=db.VDA  BreakpointsForDimension2=db.VALPHA  Table=db.CRDAR  InternalRulePriority=Speed  RndMeth=Simplest
      settings: InputPortMap=u0,u1
  CRDFL - DF,ALPHA : Lookup_n-D  BreakpointsForDimension1=db.VDF  BreakpointsForDimension2=db.VALPHA  Table=db.CRDFL  InternalRulePriority=Speed  RndMeth=Simplest
      settings: InputPortMap=u0,u1
  CRDFR - DF,ALPHA : Lookup_n-D  BreakpointsForDimension1=db.VDF  BreakpointsForDimension2=db.VALPHA  Table=db.CRDFR  InternalRulePriority=Speed  RndMeth=Simplest
      settings: InputPortMap=u0,u1
  CRDR - DR,ALPHA : Lookup_n-D  BreakpointsForDimension1=db.VDR  BreakpointsForDimension2=db.VALPHA  Table=db.CRDR  InternalRulePriority=Speed  RndMeth=Simplest
      settings: InputPortMap=u0,u1
  CRDRBETA - DR,ALPHA,BETA : Lookup_n-D  NumberOfTableDimensions=3  BreakpointsForDimension1=db.VDR  BreakpointsForDimension2=db.VALPHA  BreakpointsForDimension3=db.VBETA  Table=db.CRDRBETA  InternalRulePriority=Speed  RndMeth=Simplest
      settings: InputPortMap=u0,u1,u2
  CRHDFL - H,ALPHA,DF : Lookup_n-D  NumberOfTableDimensions=3  BreakpointsForDimension1=db.VH  BreakpointsForDimension2=db.VALPHA  BreakpointsForDimension3=db.VDF  Table=db.CRHDFL  InternalRulePriority=Speed  RndMeth=Simplest
      settings: InputPortMap=u0,u1,u2
  CRHDFR - H,ALPHA,DF : Lookup_n-D  NumberOfTableDimensions=3  BreakpointsForDimension1=db.VH  BreakpointsForDimension2=db.VALPHA  BreakpointsForDimension3=db.VDF  Table=db.CRHDFR  InternalRulePriority=Speed  RndMeth=Simplest
      settings: InputPortMap=u0,u1,u2
  Sum : Sum  Inputs=9
  CR : Outport
  wires:
  CRHDFR - H,ALPHA,DF/1 -> Sum/9  "CRHDFR"
  BusElementIn7/1 -> CRHDFL - H,ALPHA,DF/3, CRHDFR - H,ALPHA,DF/3
  CRHDFL - H,ALPHA,DF/1 -> Sum/8  "CRHDFL"
  BusElementIn6/1 -> CRHDFL - H,ALPHA,DF/1, CRHDFR - H,ALPHA,DF/1
  BusElementIn1/1 -> CRDRBETA - DR,ALPHA,BETA/3
  CRDRBETA - DR,ALPHA,BETA/1 -> Sum/7  "CRDRBETA"
  Sum/1 -> CR/1  "CR"
  BusElementIn5/1 -> CRDR - DR,ALPHA/1, CRDRBETA - DR,ALPHA,BETA/1
  CRDR - DR,ALPHA/1 -> Sum/6  "CRDR"
  CRDAR - DA,ALPHA/1 -> Sum/5  "CRDAR"
  BusElementIn3/1 -> CRDAL - DA,ALPHA/1, CRDAR - DA,ALPHA/1
  CRDAL - DA,ALPHA/1 -> Sum/4  "CRDAL"
  CRDFR - DF,ALPHA/1 -> Sum/3  "CRDFR"
  CRDFL - DF,ALPHA/1 -> Sum/2  "CRDFL"
  BusElementIn2/1 -> CRDFL - DF,ALPHA/1, CRDFR - DF,ALPHA/1
  CRBETA - BETA,ALPHA/1 -> Sum/1  "CRBETA"
  BusElementIn/1 -> CRBETA - BETA,ALPHA/2, CRDFL - DF,ALPHA/2, CRDFR - DF,ALPHA/2, CRDAL - DA,ALPHA/2, CRDAR - DA,ALPHA/2, CRDR - DR,ALPHA/2, CRDRBETA - DR,ALPHA,BETA/2, CRHDFL - H,ALPHA,DF/2, CRHDFR - H,ALPHA,DF/2
  BusElementIn8/1 -> CRBETA - BETA,ALPHA/1

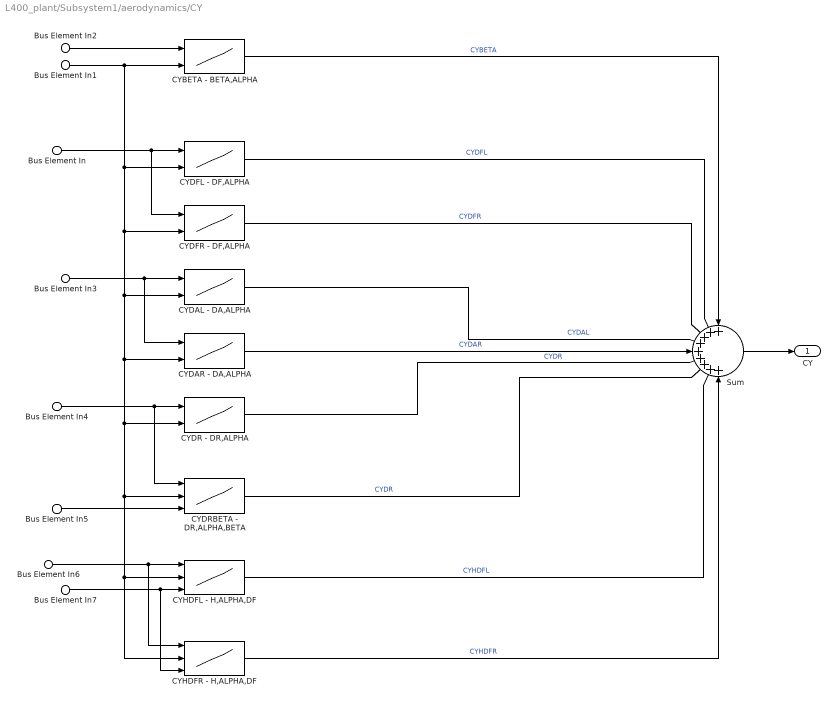
== system L400_plant/Subsystem1/aerodynamics/CY ==
  Bus Element In : Inport  PortName=cmd  Element=df
  Bus Element In7 : Inport  PortName=cmd  Element=df
  Bus Element In3 : Inport  PortName=cmd  Element=da
  Bus Element In4 : Inport  PortName=cmd  Element=dr
  Bus Element In1 : Inport  Port=2  PortName=state  Element=alpha
  Bus Element In6 : Inport  Port=2  PortName=state  Element=height
  Bus Element In2 : Inport  Port=2  PortName=state  Element=vn_ve_vd
  Bus Element In5 : Inport  Port=2  PortName=state  Element=vn_ve_vd
  CYBETA - BETA,ALPHA : Lookup_n-D  BreakpointsForDimension1=db.VBETA  BreakpointsForDimension2=db.VALPHA  Table=db.CYBETA  InternalRulePriority=Speed  RndMeth=Simplest
      settings: InputPortMap=u0,u1
  CYDAL - DA,ALPHA : Lookup_n-D  BreakpointsForDimension1=db.VDA  BreakpointsForDimension2=db.VALPHA  Table=db.CYDAL  InternalRulePriority=Speed  RndMeth=Simplest
      settings: InputPortMap=u0,u1
  CYDAR - DA,ALPHA : Lookup_n-D  BreakpointsForDimension1=db.VDA  BreakpointsForDimension2=db.VALPHA  Table=db.CYDAR  InternalRulePriority=Speed  RndMeth=Simplest
      settings: InputPortMap=u0,u1
  CYDFL - DF,ALPHA : Lookup_n-D  BreakpointsForDimension1=db.VDF  BreakpointsForDimension2=db.VALPHA  Table=db.CYDFL  InternalRulePriority=Speed  RndMeth=Simplest
      settings: InputPortMap=u0,u1
  CYDFR - DF,ALPHA : Lookup_n-D  BreakpointsForDimension1=db.VDF  BreakpointsForDimension2=db.VALPHA  Table=db.CYDFR  InternalRulePriority=Speed  RndMeth=Simplest
      settings: InputPortMap=u0,u1
  CYDR - DR,ALPHA : Lookup_n-D  BreakpointsForDimension1=db.VDR  BreakpointsForDimension2=db.VALPHA  Table=db.CYDR  InternalRulePriority=Speed  RndMeth=Simplest
      settings: InputPortMap=u0,u1
  CYDRBETA - DR,ALPHA,BETA : Lookup_n-D  NumberOfTableDimensions=3  BreakpointsForDimension1=db.VDR  BreakpointsForDimension2=db.VALPHA  BreakpointsForDimension3=db.VBETA  Table=db.CYDRBETA  InternalRulePriority=Speed  RndMeth=Simplest
      settings: InputPortMap=u0,u1,u2
  CYHDFL - H,ALPHA,DF : Lookup_n-D  NumberOfTableDimensions=3  BreakpointsForDimension1=db.VH  BreakpointsForDimension2=db.VALPHA  BreakpointsForDimension3=db.VDF  Table=db.CYHDFL  InternalRulePriority=Speed  RndMeth=Simplest
      settings: InputPortMap=u0,u1,u2
  CYHDFR - H,ALPHA,DF : Lookup_n-D  NumberOfTableDimensions=3  BreakpointsForDimension1=db.VH  BreakpointsForDimension2=db.VALPHA  BreakpointsForDimension3=db.VDF  Table=db.CYHDFR  InternalRulePriority=Speed  RndMeth=Simplest
      settings: InputPortMap=u0,u1,u2
  Sum : Sum  Inputs=9
  CY : Outport
  wires:
  Sum/1 -> CY/1
  CYBETA - BETA,ALPHA/1 -> Sum/1  "CYBETA"
  Bus Element In1/1 -> CYHDFR - H,ALPHA,DF/2, CYHDFL - H,ALPHA,DF/2, CYDRBETA - DR,ALPHA,BETA/2, CYDR - DR,ALPHA/2, CYDAR - DA,ALPHA/2, CYDAL - DA,ALPHA/2, CYDFR - DF,ALPHA/2, CYDFL - DF,ALPHA/2, CYBETA - BETA,ALPHA/2
  Bus Element In2/1 -> CYBETA - BETA,ALPHA/1
  CYDFL - DF,ALPHA/1 -> Sum/2  "CYDFL"
  Bus Element In/1 -> CYDFR - DF,ALPHA/1, CYDFL - DF,ALPHA/1
  CYDFR - DF,ALPHA/1 -> Sum/3  "CYDFR"
  CYDAL - DA,ALPHA/1 -> Sum/4  "CYDAL"
  Bus Element In3/1 -> CYDAR - DA,ALPHA/1, CYDAL - DA,ALPHA/1
  CYDAR - DA,ALPHA/1 -> Sum/5  "CYDAR"
  CYDR - DR,ALPHA/1 -> Sum/6  "CYDR"
  Bus Element In4/1 -> CYDRBETA - DR,ALPHA,BETA/1, CYDR - DR,ALPHA/1
  CYDRBETA - DR,ALPHA,BETA/1 -> Sum/7  "CYDR"
  Bus Element In5/1 -> CYDRBETA - DR,ALPHA,BETA/3
  CYHDFL - H,ALPHA,DF/1 -> Sum/8  "CYHDFL"
  Bus Element In6/1 -> CYHDFR - H,ALPHA,DF/1, CYHDFL - H,ALPHA,DF/1
  Bus Element In7/1 -> CYHDFR - H,ALPHA,DF/3, CYHDFL - H,ALPHA,DF/3
  CYHDFR - H,ALPHA,DF/1 -> Sum/9  "CYHDFR"

== system L400_plant/Subsystem1/propulsion/Subsystem ==
  In1 : Inport
  ρ : Inport  Port=2
  esc : Subsystem
  motor : Subsystem
  propeller : Subsystem
  Out1 : Outport
  Ie : Outport  Port=2
  wires:
  In1/1 -> Out1/1
  propeller/2(Torque) -> motor/3(Mload)
  motor/1(rpm) -> propeller/1(rpm)
  ρ/1 -> propeller/2(rho)
  esc/1(Um) -> motor/1(Um)
  esc/2(Ie) -> Ie/1

== system L400_plant/Subsystem1/propulsion/Subsystem/esc ==
  In1 : Inport
  Um : Outport
  Ie : Outport  Port=2
  wires:
  In1/1 -> Um/1

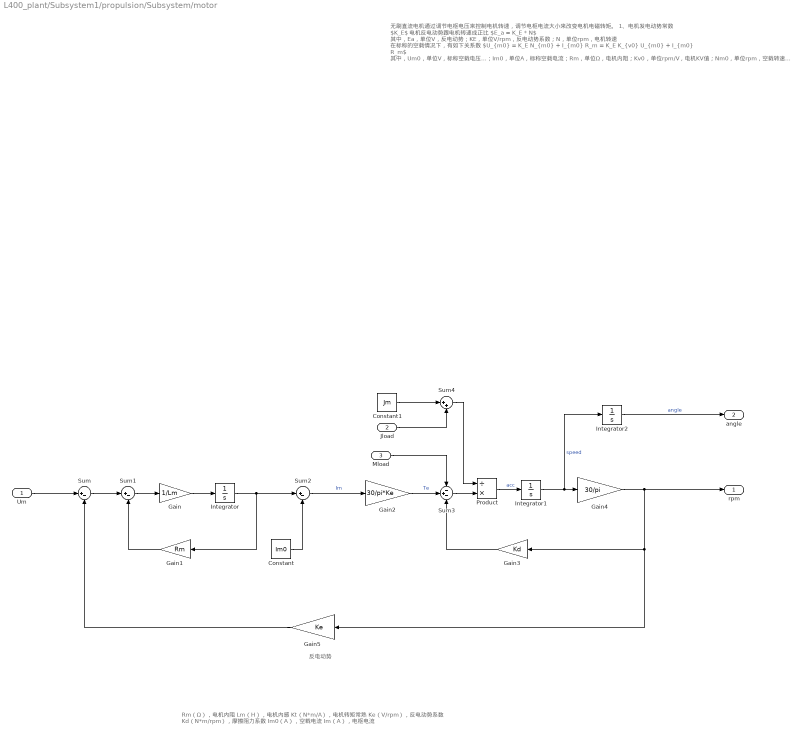
== system L400_plant/Subsystem1/propulsion/Subsystem/motor ==
  note: Rm（Ω），电机内阻
      | Lm（H），电机内感
      | Kt（N*m/A），电机转矩常熟
      | Ke（V/rpm），反电动势系数
      | Kd（N*m/rpm），摩擦阻力系数
      | Im0（A），空载电流
      | Im（A），电枢电流
  note: 反电动势
  note: 无刷直流电机通过调节电枢电压来控制电机转速，调节电枢电流大小来改变电机电磁转矩。
      |
      | 1、电机发电动势常数 $K_E$
      | 电机反电动势跟电机转速成正比
      | $E_a = K_E * N$
      | 其中，Ea，单位V，反电动势；KE，单位V/rpm，反电动势系数；N，单位rpm，电机转速
      |
      | 在标称的空载情况下，有如下关系数
      | $U_{m0} = K_E N_{m0} + I_{m0} R_m = K_E K_{v0} U_{m0} + I_{m0} R_m$
      | 其中，Um0，单位V，标称空载电压；Im0，单位A，标称空载电流；Rm，单位Ω，电机内阻；Kv0，单位rpm/V，电机KV值；Nm0，单位rpm，空载转速
      |
      | 因此可以得到反电动势常数，如下
      | $K_E = (U_{m0}-I_{m0}R_m)/(K_{v0}U_{m0})$
      |
      | 2、电机转矩常数 $K_T$
      | 电机的电磁转矩Te与电枢电流Im成正比，即
      | $T_e = K_T * I_m$
      | 电机转矩常数和发电动势常数有如下关系
      | $K_T=30K_E/pi$
      |
      | 3、电机空载电流 $I_{0}$
      | 在实际计算过程，对多旋翼无人机来说，电机空载电流和标称空载电流Im0差别不大，为了简单起见可以使用Im0表示
  Um : Inport
  Jload : Inport  Port=2
  Mload : Inport  Port=3
  Constant : Constant  Value=Im0
  Constant1 : Constant  Value=Jm
  Gain : Gain  Gain=1/Lm
  Gain1 : Gain  Gain=Rm
  Gain2 : Gain  Gain=30/pi*Ke
  Gain3 : Gain  Gain=Kd
  Gain4 : Gain  Gain=30/pi
  Gain5 : Gain  Gain=Ke
  Integrator : Integrator  LimitOutput=on
  Integrator1 : Integrator  LimitOutput=on
  Integrator2 : Integrator  WrapState=on
  Product : Product  Inputs=/*
  Sum : Sum  Inputs=|+-
  Sum1 : Sum  Inputs=|+-
  Sum2 : Sum  Inputs=|+-
  Sum3 : Sum  Inputs=-+-
  Sum4 : Sum  Inputs=|++
  rpm : Outport
  angle : Outport  Port=2
  wires:
  Um/1 -> Sum/1
  Sum/1 -> Sum1/1
  Integrator/1 -> Sum2/1, Gain1/1
  Sum1/1 -> Gain/1
  Gain/1 -> Integrator/1
  Gain1/1 -> Sum1/2
  Constant/1 -> Sum2/2
  Sum2/1 -> Gain2/1  "Im"
  Gain2/1 -> Sum3/2  "Te"
  Sum3/1 -> Product/2
  Integrator1/1 -> Integrator2/1, Gain4/1  "speed"
  Gain3/1 -> Sum3/3
  Mload/1 -> Sum3/1
  Gain4/1 -> Gain5/1, Gain3/1, rpm/1
  Product/1 -> Integrator1/1  "acc"
  Sum4/1 -> Product/1
  Constant1/1 -> Sum4/1
  Gain5/1 -> Sum/2
  Jload/1 -> Sum4/2
  Integrator2/1 -> angle/1  "angle"

== system L400_plant/Subsystem1/propulsion/Subsystem/propeller ==
  rpm : Inport  Unit=rpm
  rho : Inport  Port=2  Unit=kg/m^3
  Thrust : Outport
  Torque : Outport  Port=2
  wires:
  rpm/1 -> Thrust/1
